simulink model "Battery_Pack_Subsystem"  (R2015a)
settings: Solver=ode45  StartTime=0.0  StopTime=300  RelTol=1e-3
libraries: fl_lib x316, nesl_utility x2
(part 2 of 2)

== system Battery_Pack_Subsystem/Battery Pack/Cell50 ==
  Capacitor : fl_lib/Electrical/Electrical Elements/Capacitor  c=5000 F  r=1e-6 Ohm  g=0 1/Ohm  i_specify=off  i_priority=High  i=0 A  v_specify=off  v_priority=High  v=0 V  vc_specify=off  vc_priority=High  vc=0 V
  DC Voltage Source : fl_lib/Electrical/Electrical Sources/DC Voltage Source  v0=4 V
  Resistor : fl_lib/Electrical/Electrical Elements/Resistor  R=0.005 Ohm  i_specify=off  i_priority=High  i=0 A  v_specify=off  v_priority=High  v=0 V
  Resistor1 : fl_lib/Electrical/Electrical Elements/Resistor  R=0.1 Ohm  i_specify=off  i_priority=High  i=0 A  v_specify=off  v_priority=High  v=0 V
  - : PMIOPort  Port=1  Side=Left
  + : PMIOPort  Port=2  Side=Right
  connections:
  Capacitor/LConn1 -- Resistor/LConn1 -- Resistor1/RConn1
  Resistor/RConn1 -- Capacitor/RConn1 -- +/RConn1
  DC Voltage Source/LConn1 -- Resistor1/LConn1
  -/RConn1 -- DC Voltage Source/RConn1

== system Battery_Pack_Subsystem/Battery Pack/Cell51 ==
  Capacitor : fl_lib/Electrical/Electrical Elements/Capacitor  c=5000 F  r=1e-6 Ohm  g=0 1/Ohm  i_specify=off  i_priority=High  i=0 A  v_specify=off  v_priority=High  v=0 V  vc_specify=off  vc_priority=High  vc=0 V
  DC Voltage Source : fl_lib/Electrical/Electrical Sources/DC Voltage Source  v0=4 V
  Resistor : fl_lib/Electrical/Electrical Elements/Resistor  R=0.005 Ohm  i_specify=off  i_priority=High  i=0 A  v_specify=off  v_priority=High  v=0 V
  Resistor1 : fl_lib/Electrical/Electrical Elements/Resistor  R=0.1 Ohm  i_specify=off  i_priority=High  i=0 A  v_specify=off  v_priority=High  v=0 V
  - : PMIOPort  Port=1  Side=Left
  + : PMIOPort  Port=2  Side=Right
  connections:
  Capacitor/LConn1 -- Resistor/LConn1 -- Resistor1/RConn1
  Resistor/RConn1 -- Capacitor/RConn1 -- +/RConn1
  DC Voltage Source/LConn1 -- Resistor1/LConn1
  -/RConn1 -- DC Voltage Source/RConn1

== system Battery_Pack_Subsystem/Battery Pack/Cell52 ==
  Capacitor : fl_lib/Electrical/Electrical Elements/Capacitor  c=5000 F  r=1e-6 Ohm  g=0 1/Ohm  i_specify=off  i_priority=High  i=0 A  v_specify=off  v_priority=High  v=0 V  vc_specify=off  vc_priority=High  vc=0 V
  DC Voltage Source : fl_lib/Electrical/Electrical Sources/DC Voltage Source  v0=4 V
  Resistor : fl_lib/Electrical/Electrical Elements/Resistor  R=0.005 Ohm  i_specify=off  i_priority=High  i=0 A  v_specify=off  v_priority=High  v=0 V
  Resistor1 : fl_lib/Electrical/Electrical Elements/Resistor  R=0.1 Ohm  i_specify=off  i_priority=High  i=0 A  v_specify=off  v_priority=High  v=0 V
  - : PMIOPort  Port=1  Side=Left
  + : PMIOPort  Port=2  Side=Right
  connections:
  Capacitor/LConn1 -- Resistor/LConn1 -- Resistor1/RConn1
  Resistor/RConn1 -- Capacitor/RConn1 -- +/RConn1
  DC Voltage Source/LConn1 -- Resistor1/LConn1
  -/RConn1 -- DC Voltage Source/RConn1

== system Battery_Pack_Subsystem/Battery Pack/Cell53 ==
  Capacitor : fl_lib/Electrical/Electrical Elements/Capacitor  c=5000 F  r=1e-6 Ohm  g=0 1/Ohm  i_specify=off  i_priority=High  i=0 A  v_specify=off  v_priority=High  v=0 V  vc_specify=off  vc_priority=High  vc=0 V
  DC Voltage Source : fl_lib/Electrical/Electrical Sources/DC Voltage Source  v0=4 V
  Resistor : fl_lib/Electrical/Electrical Elements/Resistor  R=0.005 Ohm  i_specify=off  i_priority=High  i=0 A  v_specify=off  v_priority=High  v=0 V
  Resistor1 : fl_lib/Electrical/Electrical Elements/Resistor  R=0.1 Ohm  i_specify=off  i_priority=High  i=0 A  v_specify=off  v_priority=High  v=0 V
  - : PMIOPort  Port=1  Side=Left
  + : PMIOPort  Port=2  Side=Right
  connections:
  Capacitor/LConn1 -- Resistor/LConn1 -- Resistor1/RConn1
  Resistor/RConn1 -- Capacitor/RConn1 -- +/RConn1
  DC Voltage Source/LConn1 -- Resistor1/LConn1
  -/RConn1 -- DC Voltage Source/RConn1

== system Battery_Pack_Subsystem/Battery Pack/Cell54 ==
  Capacitor : fl_lib/Electrical/Electrical Elements/Capacitor  c=5000 F  r=1e-6 Ohm  g=0 1/Ohm  i_specify=off  i_priority=High  i=0 A  v_specify=off  v_priority=High  v=0 V  vc_specify=off  vc_priority=High  vc=0 V
  DC Voltage Source : fl_lib/Electrical/Electrical Sources/DC Voltage Source  v0=4 V
  Resistor : fl_lib/Electrical/Electrical Elements/Resistor  R=0.005 Ohm  i_specify=off  i_priority=High  i=0 A  v_specify=off  v_priority=High  v=0 V
  Resistor1 : fl_lib/Electrical/Electrical Elements/Resistor  R=0.1 Ohm  i_specify=off  i_priority=High  i=0 A  v_specify=off  v_priority=High  v=0 V
  - : PMIOPort  Port=1  Side=Left
  + : PMIOPort  Port=2  Side=Right
  connections:
  Capacitor/LConn1 -- Resistor/LConn1 -- Resistor1/RConn1
  Resistor/RConn1 -- Capacitor/RConn1 -- +/RConn1
  DC Voltage Source/LConn1 -- Resistor1/LConn1
  -/RConn1 -- DC Voltage Source/RConn1

== system Battery_Pack_Subsystem/Battery Pack/Cell55 ==
  Capacitor : fl_lib/Electrical/Electrical Elements/Capacitor  c=5000 F  r=1e-6 Ohm  g=0 1/Ohm  i_specify=off  i_priority=High  i=0 A  v_specify=off  v_priority=High  v=0 V  vc_specify=off  vc_priority=High  vc=0 V
  DC Voltage Source : fl_lib/Electrical/Electrical Sources/DC Voltage Source  v0=4 V
  Resistor : fl_lib/Electrical/Electrical Elements/Resistor  R=0.005 Ohm  i_specify=off  i_priority=High  i=0 A  v_specify=off  v_priority=High  v=0 V
  Resistor1 : fl_lib/Electrical/Electrical Elements/Resistor  R=0.1 Ohm  i_specify=off  i_priority=High  i=0 A  v_specify=off  v_priority=High  v=0 V
  - : PMIOPort  Port=1  Side=Left
  + : PMIOPort  Port=2  Side=Right
  connections:
  Capacitor/LConn1 -- Resistor/LConn1 -- Resistor1/RConn1
  Resistor/RConn1 -- Capacitor/RConn1 -- +/RConn1
  DC Voltage Source/LConn1 -- Resistor1/LConn1
  -/RConn1 -- DC Voltage Source/RConn1

== system Battery_Pack_Subsystem/Battery Pack/Cell56 ==
  Capacitor : fl_lib/Electrical/Electrical Elements/Capacitor  c=5000 F  r=1e-6 Ohm  g=0 1/Ohm  i_specify=off  i_priority=High  i=0 A  v_specify=off  v_priority=High  v=0 V  vc_specify=off  vc_priority=High  vc=0 V
  DC Voltage Source : fl_lib/Electrical/Electrical Sources/DC Voltage Source  v0=4 V
  Resistor : fl_lib/Electrical/Electrical Elements/Resistor  R=0.005 Ohm  i_specify=off  i_priority=High  i=0 A  v_specify=off  v_priority=High  v=0 V
  Resistor1 : fl_lib/Electrical/Electrical Elements/Resistor  R=0.1 Ohm  i_specify=off  i_priority=High  i=0 A  v_specify=off  v_priority=High  v=0 V
  - : PMIOPort  Port=1  Side=Left
  + : PMIOPort  Port=2  Side=Right
  connections:
  Capacitor/LConn1 -- Resistor/LConn1 -- Resistor1/RConn1
  Resistor/RConn1 -- Capacitor/RConn1 -- +/RConn1
  DC Voltage Source/LConn1 -- Resistor1/LConn1
  -/RConn1 -- DC Voltage Source/RConn1

== system Battery_Pack_Subsystem/Battery Pack/Cell57 ==
  Capacitor : fl_lib/Electrical/Electrical Elements/Capacitor  c=5000 F  r=1e-6 Ohm  g=0 1/Ohm  i_specify=off  i_priority=High  i=0 A  v_specify=off  v_priority=High  v=0 V  vc_specify=off  vc_priority=High  vc=0 V
  DC Voltage Source : fl_lib/Electrical/Electrical Sources/DC Voltage Source  v0=4 V
  Resistor : fl_lib/Electrical/Electrical Elements/Resistor  R=0.005 Ohm  i_specify=off  i_priority=High  i=0 A  v_specify=off  v_priority=High  v=0 V
  Resistor1 : fl_lib/Electrical/Electrical Elements/Resistor  R=0.1 Ohm  i_specify=off  i_priority=High  i=0 A  v_specify=off  v_priority=High  v=0 V
  - : PMIOPort  Port=1  Side=Left
  + : PMIOPort  Port=2  Side=Right
  connections:
  Capacitor/LConn1 -- Resistor/LConn1 -- Resistor1/RConn1
  Resistor/RConn1 -- Capacitor/RConn1 -- +/RConn1
  DC Voltage Source/LConn1 -- Resistor1/LConn1
  -/RConn1 -- DC Voltage Source/RConn1

== system Battery_Pack_Subsystem/Battery Pack/Cell58 ==
  Capacitor : fl_lib/Electrical/Electrical Elements/Capacitor  c=5000 F  r=1e-6 Ohm  g=0 1/Ohm  i_specify=off  i_priority=High  i=0 A  v_specify=off  v_priority=High  v=0 V  vc_specify=off  vc_priority=High  vc=0 V
  DC Voltage Source : fl_lib/Electrical/Electrical Sources/DC Voltage Source  v0=4 V
  Resistor : fl_lib/Electrical/Electrical Elements/Resistor  R=0.005 Ohm  i_specify=off  i_priority=High  i=0 A  v_specify=off  v_priority=High  v=0 V
  Resistor1 : fl_lib/Electrical/Electrical Elements/Resistor  R=0.1 Ohm  i_specify=off  i_priority=High  i=0 A  v_specify=off  v_priority=High  v=0 V
  - : PMIOPort  Port=1  Side=Left
  + : PMIOPort  Port=2  Side=Right
  connections:
  Capacitor/LConn1 -- Resistor/LConn1 -- Resistor1/RConn1
  Resistor/RConn1 -- Capacitor/RConn1 -- +/RConn1
  DC Voltage Source/LConn1 -- Resistor1/LConn1
  -/RConn1 -- DC Voltage Source/RConn1

== system Battery_Pack_Subsystem/Battery Pack/Cell59 ==
  Capacitor : fl_lib/Electrical/Electrical Elements/Capacitor  c=5000 F  r=1e-6 Ohm  g=0 1/Ohm  i_specify=off  i_priority=High  i=0 A  v_specify=off  v_priority=High  v=0 V  vc_specify=off  vc_priority=High  vc=0 V
  DC Voltage Source : fl_lib/Electrical/Electrical Sources/DC Voltage Source  v0=4 V
  Resistor : fl_lib/Electrical/Electrical Elements/Resistor  R=0.005 Ohm  i_specify=off  i_priority=High  i=0 A  v_specify=off  v_priority=High  v=0 V
  Resistor1 : fl_lib/Electrical/Electrical Elements/Resistor  R=0.1 Ohm  i_specify=off  i_priority=High  i=0 A  v_specify=off  v_priority=High  v=0 V
  - : PMIOPort  Port=1  Side=Left
  + : PMIOPort  Port=2  Side=Right
  connections:
  Capacitor/LConn1 -- Resistor/LConn1 -- Resistor1/RConn1
  Resistor/RConn1 -- Capacitor/RConn1 -- +/RConn1
  DC Voltage Source/LConn1 -- Resistor1/LConn1
  -/RConn1 -- DC Voltage Source/RConn1

== system Battery_Pack_Subsystem/Battery Pack/Cell6 ==
  Capacitor : fl_lib/Electrical/Electrical Elements/Capacitor  c=5000 F  r=1e-6 Ohm  g=0 1/Ohm  i_specify=off  i_priority=High  i=0 A  v_specify=off  v_priority=High  v=0 V  vc_specify=off  vc_priority=High  vc=0 V
  DC Voltage Source : fl_lib/Electrical/Electrical Sources/DC Voltage Source  v0=4 V
  Resistor : fl_lib/Electrical/Electrical Elements/Resistor  R=0.005 Ohm  i_specify=off  i_priority=High  i=0 A  v_specify=off  v_priority=High  v=0 V
  Resistor1 : fl_lib/Electrical/Electrical Elements/Resistor  R=0.1 Ohm  i_specify=off  i_priority=High  i=0 A  v_specify=off  v_priority=High  v=0 V
  - : PMIOPort  Port=1  Side=Left
  + : PMIOPort  Port=2  Side=Right
  connections:
  Capacitor/LConn1 -- Resistor/LConn1 -- Resistor1/RConn1
  Resistor/RConn1 -- Capacitor/RConn1 -- +/RConn1
  DC Voltage Source/LConn1 -- Resistor1/LConn1
  -/RConn1 -- DC Voltage Source/RConn1

== system Battery_Pack_Subsystem/Battery Pack/Cell60 ==
  Capacitor : fl_lib/Electrical/Electrical Elements/Capacitor  c=5000 F  r=1e-6 Ohm  g=0 1/Ohm  i_specify=off  i_priority=High  i=0 A  v_specify=off  v_priority=High  v=0 V  vc_specify=off  vc_priority=High  vc=0 V
  DC Voltage Source : fl_lib/Electrical/Electrical Sources/DC Voltage Source  v0=4 V
  Resistor : fl_lib/Electrical/Electrical Elements/Resistor  R=0.005 Ohm  i_specify=off  i_priority=High  i=0 A  v_specify=off  v_priority=High  v=0 V
  Resistor1 : fl_lib/Electrical/Electrical Elements/Resistor  R=0.1 Ohm  i_specify=off  i_priority=High  i=0 A  v_specify=off  v_priority=High  v=0 V
  - : PMIOPort  Port=1  Side=Left
  + : PMIOPort  Port=2  Side=Right
  connections:
  Capacitor/LConn1 -- Resistor/LConn1 -- Resistor1/RConn1
  Resistor/RConn1 -- Capacitor/RConn1 -- +/RConn1
  DC Voltage Source/LConn1 -- Resistor1/LConn1
  -/RConn1 -- DC Voltage Source/RConn1

== system Battery_Pack_Subsystem/Battery Pack/Cell61 ==
  Capacitor : fl_lib/Electrical/Electrical Elements/Capacitor  c=5000 F  r=1e-6 Ohm  g=0 1/Ohm  i_specify=off  i_priority=High  i=0 A  v_specify=off  v_priority=High  v=0 V  vc_specify=off  vc_priority=High  vc=0 V
  DC Voltage Source : fl_lib/Electrical/Electrical Sources/DC Voltage Source  v0=4 V
  Resistor : fl_lib/Electrical/Electrical Elements/Resistor  R=0.005 Ohm  i_specify=off  i_priority=High  i=0 A  v_specify=off  v_priority=High  v=0 V
  Resistor1 : fl_lib/Electrical/Electrical Elements/Resistor  R=0.1 Ohm  i_specify=off  i_priority=High  i=0 A  v_specify=off  v_priority=High  v=0 V
  - : PMIOPort  Port=1  Side=Left
  + : PMIOPort  Port=2  Side=Right
  connections:
  Capacitor/LConn1 -- Resistor/LConn1 -- Resistor1/RConn1
  Resistor/RConn1 -- Capacitor/RConn1 -- +/RConn1
  DC Voltage Source/LConn1 -- Resistor1/LConn1
  -/RConn1 -- DC Voltage Source/RConn1

== system Battery_Pack_Subsystem/Battery Pack/Cell62 ==
  Capacitor : fl_lib/Electrical/Electrical Elements/Capacitor  c=5000 F  r=1e-6 Ohm  g=0 1/Ohm  i_specify=off  i_priority=High  i=0 A  v_specify=off  v_priority=High  v=0 V  vc_specify=off  vc_priority=High  vc=0 V
  DC Voltage Source : fl_lib/Electrical/Electrical Sources/DC Voltage Source  v0=4 V
  Resistor : fl_lib/Electrical/Electrical Elements/Resistor  R=0.005 Ohm  i_specify=off  i_priority=High  i=0 A  v_specify=off  v_priority=High  v=0 V
  Resistor1 : fl_lib/Electrical/Electrical Elements/Resistor  R=0.1 Ohm  i_specify=off  i_priority=High  i=0 A  v_specify=off  v_priority=High  v=0 V
  - : PMIOPort  Port=1  Side=Left
  + : PMIOPort  Port=2  Side=Right
  connections:
  Capacitor/LConn1 -- Resistor/LConn1 -- Resistor1/RConn1
  Resistor/RConn1 -- Capacitor/RConn1 -- +/RConn1
  DC Voltage Source/LConn1 -- Resistor1/LConn1
  -/RConn1 -- DC Voltage Source/RConn1

== system Battery_Pack_Subsystem/Battery Pack/Cell63 ==
  Capacitor : fl_lib/Electrical/Electrical Elements/Capacitor  c=5000 F  r=1e-6 Ohm  g=0 1/Ohm  i_specify=off  i_priority=High  i=0 A  v_specify=off  v_priority=High  v=0 V  vc_specify=off  vc_priority=High  vc=0 V
  DC Voltage Source : fl_lib/Electrical/Electrical Sources/DC Voltage Source  v0=4 V
  Resistor : fl_lib/Electrical/Electrical Elements/Resistor  R=0.005 Ohm  i_specify=off  i_priority=High  i=0 A  v_specify=off  v_priority=High  v=0 V
  Resistor1 : fl_lib/Electrical/Electrical Elements/Resistor  R=0.1 Ohm  i_specify=off  i_priority=High  i=0 A  v_specify=off  v_priority=High  v=0 V
  - : PMIOPort  Port=1  Side=Left
  + : PMIOPort  Port=2  Side=Right
  connections:
  Capacitor/LConn1 -- Resistor/LConn1 -- Resistor1/RConn1
  Resistor/RConn1 -- Capacitor/RConn1 -- +/RConn1
  DC Voltage Source/LConn1 -- Resistor1/LConn1
  -/RConn1 -- DC Voltage Source/RConn1

== system Battery_Pack_Subsystem/Battery Pack/Cell64 ==
  Capacitor : fl_lib/Electrical/Electrical Elements/Capacitor  c=5000 F  r=1e-6 Ohm  g=0 1/Ohm  i_specify=off  i_priority=High  i=0 A  v_specify=off  v_priority=High  v=0 V  vc_specify=off  vc_priority=High  vc=0 V
  DC Voltage Source : fl_lib/Electrical/Electrical Sources/DC Voltage Source  v0=4 V
  Resistor : fl_lib/Electrical/Electrical Elements/Resistor  R=0.005 Ohm  i_specify=off  i_priority=High  i=0 A  v_specify=off  v_priority=High  v=0 V
  Resistor1 : fl_lib/Electrical/Electrical Elements/Resistor  R=0.1 Ohm  i_specify=off  i_priority=High  i=0 A  v_specify=off  v_priority=High  v=0 V
  - : PMIOPort  Port=1  Side=Left
  + : PMIOPort  Port=2  Side=Right
  connections:
  Capacitor/LConn1 -- Resistor/LConn1 -- Resistor1/RConn1
  Resistor/RConn1 -- Capacitor/RConn1 -- +/RConn1
  DC Voltage Source/LConn1 -- Resistor1/LConn1
  -/RConn1 -- DC Voltage Source/RConn1

== system Battery_Pack_Subsystem/Battery Pack/Cell65 ==
  Capacitor : fl_lib/Electrical/Electrical Elements/Capacitor  c=5000 F  r=1e-6 Ohm  g=0 1/Ohm  i_specify=off  i_priority=High  i=0 A  v_specify=off  v_priority=High  v=0 V  vc_specify=off  vc_priority=High  vc=0 V
  DC Voltage Source : fl_lib/Electrical/Electrical Sources/DC Voltage Source  v0=4 V
  Resistor : fl_lib/Electrical/Electrical Elements/Resistor  R=0.005 Ohm  i_specify=off  i_priority=High  i=0 A  v_specify=off  v_priority=High  v=0 V
  Resistor1 : fl_lib/Electrical/Electrical Elements/Resistor  R=0.1 Ohm  i_specify=off  i_priority=High  i=0 A  v_specify=off  v_priority=High  v=0 V
  - : PMIOPort  Port=1  Side=Left
  + : PMIOPort  Port=2  Side=Right
  connections:
  Capacitor/LConn1 -- Resistor/LConn1 -- Resistor1/RConn1
  Resistor/RConn1 -- Capacitor/RConn1 -- +/RConn1
  DC Voltage Source/LConn1 -- Resistor1/LConn1
  -/RConn1 -- DC Voltage Source/RConn1

== system Battery_Pack_Subsystem/Battery Pack/Cell66 ==
  Capacitor : fl_lib/Electrical/Electrical Elements/Capacitor  c=5000 F  r=1e-6 Ohm  g=0 1/Ohm  i_specify=off  i_priority=High  i=0 A  v_specify=off  v_priority=High  v=0 V  vc_specify=off  vc_priority=High  vc=0 V
  DC Voltage Source : fl_lib/Electrical/Electrical Sources/DC Voltage Source  v0=4 V
  Resistor : fl_lib/Electrical/Electrical Elements/Resistor  R=0.005 Ohm  i_specify=off  i_priority=High  i=0 A  v_specify=off  v_priority=High  v=0 V
  Resistor1 : fl_lib/Electrical/Electrical Elements/Resistor  R=0.1 Ohm  i_specify=off  i_priority=High  i=0 A  v_specify=off  v_priority=High  v=0 V
  - : PMIOPort  Port=1  Side=Left
  + : PMIOPort  Port=2  Side=Right
  connections:
  Capacitor/LConn1 -- Resistor/LConn1 -- Resistor1/RConn1
  Resistor/RConn1 -- Capacitor/RConn1 -- +/RConn1
  DC Voltage Source/LConn1 -- Resistor1/LConn1
  -/RConn1 -- DC Voltage Source/RConn1

== system Battery_Pack_Subsystem/Battery Pack/Cell67 ==
  Capacitor : fl_lib/Electrical/Electrical Elements/Capacitor  c=5000 F  r=1e-6 Ohm  g=0 1/Ohm  i_specify=off  i_priority=High  i=0 A  v_specify=off  v_priority=High  v=0 V  vc_specify=off  vc_priority=High  vc=0 V
  DC Voltage Source : fl_lib/Electrical/Electrical Sources/DC Voltage Source  v0=4 V
  Resistor : fl_lib/Electrical/Electrical Elements/Resistor  R=0.005 Ohm  i_specify=off  i_priority=High  i=0 A  v_specify=off  v_priority=High  v=0 V
  Resistor1 : fl_lib/Electrical/Electrical Elements/Resistor  R=0.1 Ohm  i_specify=off  i_priority=High  i=0 A  v_specify=off  v_priority=High  v=0 V
  - : PMIOPort  Port=1  Side=Left
  + : PMIOPort  Port=2  Side=Right
  connections:
  Capacitor/LConn1 -- Resistor/LConn1 -- Resistor1/RConn1
  Resistor/RConn1 -- Capacitor/RConn1 -- +/RConn1
  DC Voltage Source/LConn1 -- Resistor1/LConn1
  -/RConn1 -- DC Voltage Source/RConn1

== system Battery_Pack_Subsystem/Battery Pack/Cell68 ==
  Capacitor : fl_lib/Electrical/Electrical Elements/Capacitor  c=5000 F  r=1e-6 Ohm  g=0 1/Ohm  i_specify=off  i_priority=High  i=0 A  v_specify=off  v_priority=High  v=0 V  vc_specify=off  vc_priority=High  vc=0 V
  DC Voltage Source : fl_lib/Electrical/Electrical Sources/DC Voltage Source  v0=4 V
  Resistor : fl_lib/Electrical/Electrical Elements/Resistor  R=0.005 Ohm  i_specify=off  i_priority=High  i=0 A  v_specify=off  v_priority=High  v=0 V
  Resistor1 : fl_lib/Electrical/Electrical Elements/Resistor  R=0.1 Ohm  i_specify=off  i_priority=High  i=0 A  v_specify=off  v_priority=High  v=0 V
  - : PMIOPort  Port=1  Side=Left
  + : PMIOPort  Port=2  Side=Right
  connections:
  Capacitor/LConn1 -- Resistor/LConn1 -- Resistor1/RConn1
  Resistor/RConn1 -- Capacitor/RConn1 -- +/RConn1
  DC Voltage Source/LConn1 -- Resistor1/LConn1
  -/RConn1 -- DC Voltage Source/RConn1

== system Battery_Pack_Subsystem/Battery Pack/Cell69 ==
  Capacitor : fl_lib/Electrical/Electrical Elements/Capacitor  c=5000 F  r=1e-6 Ohm  g=0 1/Ohm  i_specify=off  i_priority=High  i=0 A  v_specify=off  v_priority=High  v=0 V  vc_specify=off  vc_priority=High  vc=0 V
  DC Voltage Source : fl_lib/Electrical/Electrical Sources/DC Voltage Source  v0=4 V
  Resistor : fl_lib/Electrical/Electrical Elements/Resistor  R=0.005 Ohm  i_specify=off  i_priority=High  i=0 A  v_specify=off  v_priority=High  v=0 V
  Resistor1 : fl_lib/Electrical/Electrical Elements/Resistor  R=0.1 Ohm  i_specify=off  i_priority=High  i=0 A  v_specify=off  v_priority=High  v=0 V
  - : PMIOPort  Port=1  Side=Left
  + : PMIOPort  Port=2  Side=Right
  connections:
  Capacitor/LConn1 -- Resistor/LConn1 -- Resistor1/RConn1
  Resistor/RConn1 -- Capacitor/RConn1 -- +/RConn1
  DC Voltage Source/LConn1 -- Resistor1/LConn1
  -/RConn1 -- DC Voltage Source/RConn1

== system Battery_Pack_Subsystem/Battery Pack/Cell7 ==
  Capacitor : fl_lib/Electrical/Electrical Elements/Capacitor  c=5000 F  r=1e-6 Ohm  g=0 1/Ohm  i_specify=off  i_priority=High  i=0 A  v_specify=off  v_priority=High  v=0 V  vc_specify=off  vc_priority=High  vc=0 V
  DC Voltage Source : fl_lib/Electrical/Electrical Sources/DC Voltage Source  v0=4 V
  Resistor : fl_lib/Electrical/Electrical Elements/Resistor  R=0.005 Ohm  i_specify=off  i_priority=High  i=0 A  v_specify=off  v_priority=High  v=0 V
  Resistor1 : fl_lib/Electrical/Electrical Elements/Resistor  R=0.1 Ohm  i_specify=off  i_priority=High  i=0 A  v_specify=off  v_priority=High  v=0 V
  - : PMIOPort  Port=1  Side=Left
  + : PMIOPort  Port=2  Side=Right
  connections:
  Capacitor/LConn1 -- Resistor/LConn1 -- Resistor1/RConn1
  Resistor/RConn1 -- Capacitor/RConn1 -- +/RConn1
  DC Voltage Source/LConn1 -- Resistor1/LConn1
  -/RConn1 -- DC Voltage Source/RConn1

== system Battery_Pack_Subsystem/Battery Pack/Cell70 ==
  Capacitor : fl_lib/Electrical/Electrical Elements/Capacitor  c=5000 F  r=1e-6 Ohm  g=0 1/Ohm  i_specify=off  i_priority=High  i=0 A  v_specify=off  v_priority=High  v=0 V  vc_specify=off  vc_priority=High  vc=0 V
  DC Voltage Source : fl_lib/Electrical/Electrical Sources/DC Voltage Source  v0=4 V
  Resistor : fl_lib/Electrical/Electrical Elements/Resistor  R=0.005 Ohm  i_specify=off  i_priority=High  i=0 A  v_specify=off  v_priority=High  v=0 V
  Resistor1 : fl_lib/Electrical/Electrical Elements/Resistor  R=0.1 Ohm  i_specify=off  i_priority=High  i=0 A  v_specify=off  v_priority=High  v=0 V
  - : PMIOPort  Port=1  Side=Left
  + : PMIOPort  Port=2  Side=Right
  connections:
  Capacitor/LConn1 -- Resistor/LConn1 -- Resistor1/RConn1
  Resistor/RConn1 -- Capacitor/RConn1 -- +/RConn1
  DC Voltage Source/LConn1 -- Resistor1/LConn1
  -/RConn1 -- DC Voltage Source/RConn1

== system Battery_Pack_Subsystem/Battery Pack/Cell71 ==
  Capacitor : fl_lib/Electrical/Electrical Elements/Capacitor  c=5000 F  r=1e-6 Ohm  g=0 1/Ohm  i_specify=off  i_priority=High  i=0 A  v_specify=off  v_priority=High  v=0 V  vc_specify=off  vc_priority=High  vc=0 V
  DC Voltage Source : fl_lib/Electrical/Electrical Sources/DC Voltage Source  v0=4 V
  Resistor : fl_lib/Electrical/Electrical Elements/Resistor  R=0.005 Ohm  i_specify=off  i_priority=High  i=0 A  v_specify=off  v_priority=High  v=0 V
  Resistor1 : fl_lib/Electrical/Electrical Elements/Resistor  R=0.1 Ohm  i_specify=off  i_priority=High  i=0 A  v_specify=off  v_priority=High  v=0 V
  - : PMIOPort  Port=1  Side=Left
  + : PMIOPort  Port=2  Side=Right
  connections:
  Capacitor/LConn1 -- Resistor/LConn1 -- Resistor1/RConn1
  Resistor/RConn1 -- Capacitor/RConn1 -- +/RConn1
  DC Voltage Source/LConn1 -- Resistor1/LConn1
  -/RConn1 -- DC Voltage Source/RConn1

== system Battery_Pack_Subsystem/Battery Pack/Cell72 ==
  Capacitor : fl_lib/Electrical/Electrical Elements/Capacitor  c=5000 F  r=1e-6 Ohm  g=0 1/Ohm  i_specify=off  i_priority=High  i=0 A  v_specify=off  v_priority=High  v=0 V  vc_specify=off  vc_priority=High  vc=0 V
  DC Voltage Source : fl_lib/Electrical/Electrical Sources/DC Voltage Source  v0=4 V
  Resistor : fl_lib/Electrical/Electrical Elements/Resistor  R=0.005 Ohm  i_specify=off  i_priority=High  i=0 A  v_specify=off  v_priority=High  v=0 V
  Resistor1 : fl_lib/Electrical/Electrical Elements/Resistor  R=0.1 Ohm  i_specify=off  i_priority=High  i=0 A  v_specify=off  v_priority=High  v=0 V
  - : PMIOPort  Port=1  Side=Left
  + : PMIOPort  Port=2  Side=Right
  connections:
  Capacitor/LConn1 -- Resistor/LConn1 -- Resistor1/RConn1
  Resistor/RConn1 -- Capacitor/RConn1 -- +/RConn1
  DC Voltage Source/LConn1 -- Resistor1/LConn1
  -/RConn1 -- DC Voltage Source/RConn1

== system Battery_Pack_Subsystem/Battery Pack/Cell73 ==
  Capacitor : fl_lib/Electrical/Electrical Elements/Capacitor  c=5000 F  r=1e-6 Ohm  g=0 1/Ohm  i_specify=off  i_priority=High  i=0 A  v_specify=off  v_priority=High  v=0 V  vc_specify=off  vc_priority=High  vc=0 V
  DC Voltage Source : fl_lib/Electrical/Electrical Sources/DC Voltage Source  v0=4 V
  Resistor : fl_lib/Electrical/Electrical Elements/Resistor  R=0.005 Ohm  i_specify=off  i_priority=High  i=0 A  v_specify=off  v_priority=High  v=0 V
  Resistor1 : fl_lib/Electrical/Electrical Elements/Resistor  R=0.1 Ohm  i_specify=off  i_priority=High  i=0 A  v_specify=off  v_priority=High  v=0 V
  - : PMIOPort  Port=1  Side=Left
  + : PMIOPort  Port=2  Side=Right
  connections:
  Capacitor/LConn1 -- Resistor/LConn1 -- Resistor1/RConn1
  Resistor/RConn1 -- Capacitor/RConn1 -- +/RConn1
  DC Voltage Source/LConn1 -- Resistor1/LConn1
  -/RConn1 -- DC Voltage Source/RConn1

== system Battery_Pack_Subsystem/Battery Pack/Cell74 ==
  Capacitor : fl_lib/Electrical/Electrical Elements/Capacitor  c=5000 F  r=1e-6 Ohm  g=0 1/Ohm  i_specify=off  i_priority=High  i=0 A  v_specify=off  v_priority=High  v=0 V  vc_specify=off  vc_priority=High  vc=0 V
  DC Voltage Source : fl_lib/Electrical/Electrical Sources/DC Voltage Source  v0=4 V
  Resistor : fl_lib/Electrical/Electrical Elements/Resistor  R=0.005 Ohm  i_specify=off  i_priority=High  i=0 A  v_specify=off  v_priority=High  v=0 V
  Resistor1 : fl_lib/Electrical/Electrical Elements/Resistor  R=0.1 Ohm  i_specify=off  i_priority=High  i=0 A  v_specify=off  v_priority=High  v=0 V
  - : PMIOPort  Port=1  Side=Left
  + : PMIOPort  Port=2  Side=Right
  connections:
  Capacitor/LConn1 -- Resistor/LConn1 -- Resistor1/RConn1
  Resistor/RConn1 -- Capacitor/RConn1 -- +/RConn1
  DC Voltage Source/LConn1 -- Resistor1/LConn1
  -/RConn1 -- DC Voltage Source/RConn1

== system Battery_Pack_Subsystem/Battery Pack/Cell75 ==
  Capacitor : fl_lib/Electrical/Electrical Elements/Capacitor  c=5000 F  r=1e-6 Ohm  g=0 1/Ohm  i_specify=off  i_priority=High  i=0 A  v_specify=off  v_priority=High  v=0 V  vc_specify=off  vc_priority=High  vc=0 V
  DC Voltage Source : fl_lib/Electrical/Electrical Sources/DC Voltage Source  v0=4 V
  Resistor : fl_lib/Electrical/Electrical Elements/Resistor  R=0.005 Ohm  i_specify=off  i_priority=High  i=0 A  v_specify=off  v_priority=High  v=0 V
  Resistor1 : fl_lib/Electrical/Electrical Elements/Resistor  R=0.1 Ohm  i_specify=off  i_priority=High  i=0 A  v_specify=off  v_priority=High  v=0 V
  - : PMIOPort  Port=1  Side=Left
  + : PMIOPort  Port=2  Side=Right
  connections:
  Capacitor/LConn1 -- Resistor/LConn1 -- Resistor1/RConn1
  Resistor/RConn1 -- Capacitor/RConn1 -- +/RConn1
  DC Voltage Source/LConn1 -- Resistor1/LConn1
  -/RConn1 -- DC Voltage Source/RConn1

== system Battery_Pack_Subsystem/Battery Pack/Cell76 ==
  Capacitor : fl_lib/Electrical/Electrical Elements/Capacitor  c=5000 F  r=1e-6 Ohm  g=0 1/Ohm  i_specify=off  i_priority=High  i=0 A  v_specify=off  v_priority=High  v=0 V  vc_specify=off  vc_priority=High  vc=0 V
  DC Voltage Source : fl_lib/Electrical/Electrical Sources/DC Voltage Source  v0=4 V
  Resistor : fl_lib/Electrical/Electrical Elements/Resistor  R=0.005 Ohm  i_specify=off  i_priority=High  i=0 A  v_specify=off  v_priority=High  v=0 V
  Resistor1 : fl_lib/Electrical/Electrical Elements/Resistor  R=0.1 Ohm  i_specify=off  i_priority=High  i=0 A  v_specify=off  v_priority=High  v=0 V
  - : PMIOPort  Port=1  Side=Left
  + : PMIOPort  Port=2  Side=Right
  connections:
  Capacitor/LConn1 -- Resistor/LConn1 -- Resistor1/RConn1
  Resistor/RConn1 -- Capacitor/RConn1 -- +/RConn1
  DC Voltage Source/LConn1 -- Resistor1/LConn1
  -/RConn1 -- DC Voltage Source/RConn1

== system Battery_Pack_Subsystem/Battery Pack/Cell77 ==
  Capacitor : fl_lib/Electrical/Electrical Elements/Capacitor  c=5000 F  r=1e-6 Ohm  g=0 1/Ohm  i_specify=off  i_priority=High  i=0 A  v_specify=off  v_priority=High  v=0 V  vc_specify=off  vc_priority=High  vc=0 V
  DC Voltage Source : fl_lib/Electrical/Electrical Sources/DC Voltage Source  v0=4 V
  Resistor : fl_lib/Electrical/Electrical Elements/Resistor  R=0.005 Ohm  i_specify=off  i_priority=High  i=0 A  v_specify=off  v_priority=High  v=0 V
  Resistor1 : fl_lib/Electrical/Electrical Elements/Resistor  R=0.1 Ohm  i_specify=off  i_priority=High  i=0 A  v_specify=off  v_priority=High  v=0 V
  - : PMIOPort  Port=1  Side=Left
  + : PMIOPort  Port=2  Side=Right
  connections:
  Capacitor/LConn1 -- Resistor/LConn1 -- Resistor1/RConn1
  Resistor/RConn1 -- Capacitor/RConn1 -- +/RConn1
  DC Voltage Source/LConn1 -- Resistor1/LConn1
  -/RConn1 -- DC Voltage Source/RConn1

== system Battery_Pack_Subsystem/Battery Pack/Cell8 ==
  Capacitor : fl_lib/Electrical/Electrical Elements/Capacitor  c=5000 F  r=1e-6 Ohm  g=0 1/Ohm  i_specify=off  i_priority=High  i=0 A  v_specify=off  v_priority=High  v=0 V  vc_specify=off  vc_priority=High  vc=0 V
  DC Voltage Source : fl_lib/Electrical/Electrical Sources/DC Voltage Source  v0=4 V
  Resistor : fl_lib/Electrical/Electrical Elements/Resistor  R=0.005 Ohm  i_specify=off  i_priority=High  i=0 A  v_specify=off  v_priority=High  v=0 V
  Resistor1 : fl_lib/Electrical/Electrical Elements/Resistor  R=0.1 Ohm  i_specify=off  i_priority=High  i=0 A  v_specify=off  v_priority=High  v=0 V
  - : PMIOPort  Port=1  Side=Left
  + : PMIOPort  Port=2  Side=Right
  connections:
  Capacitor/LConn1 -- Resistor/LConn1 -- Resistor1/RConn1
  Resistor/RConn1 -- Capacitor/RConn1 -- +/RConn1
  DC Voltage Source/LConn1 -- Resistor1/LConn1
  -/RConn1 -- DC Voltage Source/RConn1

== system Battery_Pack_Subsystem/Battery Pack/Cell9 ==
  Capacitor : fl_lib/Electrical/Electrical Elements/Capacitor  c=5000 F  r=1e-6 Ohm  g=0 1/Ohm  i_specify=off  i_priority=High  i=0 A  v_specify=off  v_priority=High  v=0 V  vc_specify=off  vc_priority=High  vc=0 V
  DC Voltage Source : fl_lib/Electrical/Electrical Sources/DC Voltage Source  v0=4 V
  Resistor : fl_lib/Electrical/Electrical Elements/Resistor  R=0.005 Ohm  i_specify=off  i_priority=High  i=0 A  v_specify=off  v_priority=High  v=0 V
  Resistor1 : fl_lib/Electrical/Electrical Elements/Resistor  R=0.1 Ohm  i_specify=off  i_priority=High  i=0 A  v_specify=off  v_priority=High  v=0 V
  - : PMIOPort  Port=1  Side=Left
  + : PMIOPort  Port=2  Side=Right
  connections:
  Capacitor/LConn1 -- Resistor/LConn1 -- Resistor1/RConn1
  Resistor/RConn1 -- Capacitor/RConn1 -- +/RConn1
  DC Voltage Source/LConn1 -- Resistor1/LConn1
  -/RConn1 -- DC Voltage Source/RConn1
